simulink model "series_simulink"  (R2018a)
settings: Solver=VariableStepAuto  StartTime=0.0  StopTime=10.0  RelTol=1e-3
libraries: cstblocks x7
settings Model: Creator=muhsi  LastModifiedBy=muhsi

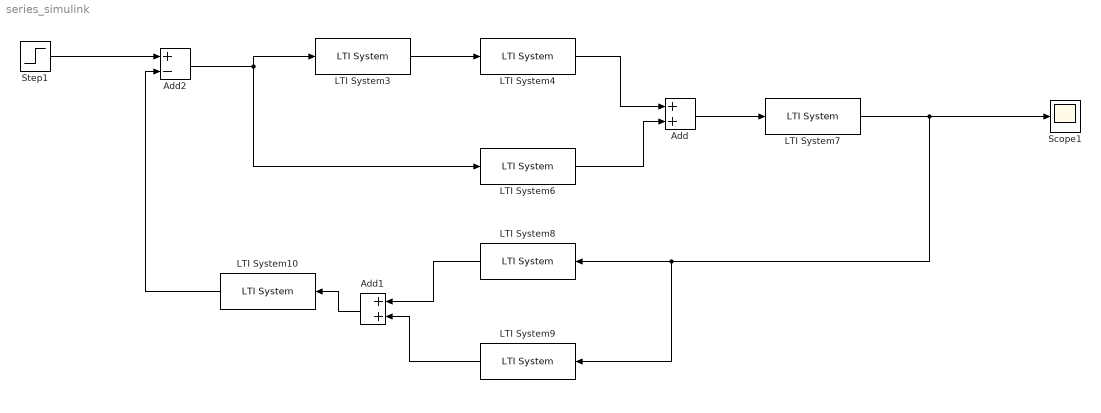
== system series_simulink ==
  Add : Sum
  Add1 : Sum
  Add2 : Sum  Inputs=+-
  LTI System10 : cstblocks/LTI System  sys=tf([1 3],[1 5])  IC=[]
  LTI System3 : cstblocks/LTI System  sys=tf(1,[1 1])  IC=[]
  LTI System4 : cstblocks/LTI System  sys=tf(1,[1 4])  IC=[]
  LTI System6 : cstblocks/LTI System  sys=tf([1 3],[1 5])  IC=[]
  LTI System7 : cstblocks/LTI System  sys=tf([1 3],[1 5])  IC=[]
  LTI System8 : cstblocks/LTI System  sys=tf(1,[1 1])  IC=[]
  LTI System9 : cstblocks/LTI System  sys=tf(1,[1 4])  IC=[]
  Scope1 : Scope
  Step1 : Step  SampleTime=0
  wires:
  LTI System3/1 -> LTI System4/1
  LTI System4/1 -> Add/1
  LTI System6/1 -> Add/2
  Add/1 -> LTI System7/1
  LTI System8/1 -> Add1/1
  LTI System9/1 -> Add1/2
  Add1/1 -> LTI System10/1
  LTI System10/1 -> Add2/2
  Step1/1 -> Add2/1
  Add2/1 -> LTI System6/1, LTI System3/1
  LTI System7/1 -> LTI System9/1, LTI System8/1, Scope1/1
